simulink model "UnrealSimulinkController"  (R2025b)
settings: Solver=VariableStepAuto  StartTime=0.0  StopTime=inf  RelTol=1e-3
libraries: sim3dlib x3
settings Model: Creator=Liam  LastModifiedBy=Liam

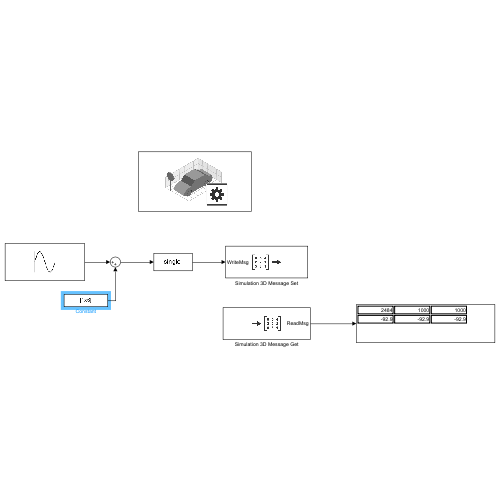
[thumbnail: Simulink's stored preview of the top-level diagram]
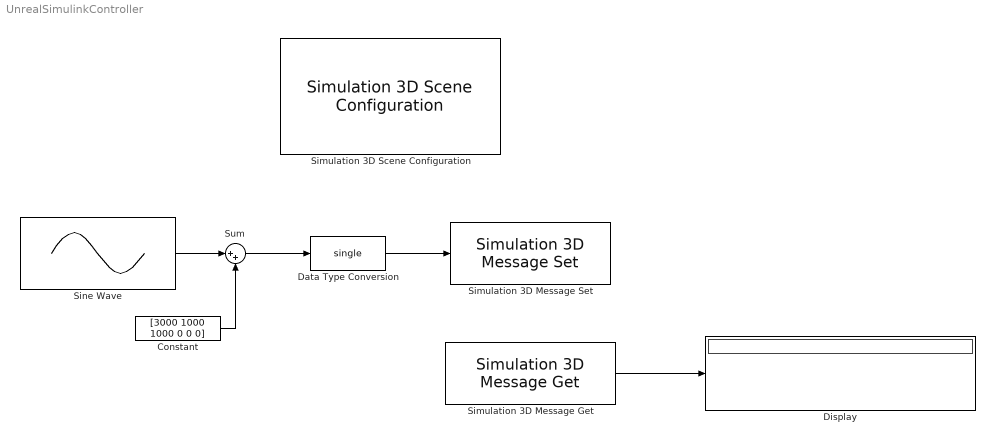
== system UnrealSimulinkController ==
  Constant : Constant  Value=[3000 1000 1000 0 0 0]  VectorParams1D=off  OutDataTypeStr=single
  Data Type Conversion : DataTypeConversion  OutDataTypeStr=single  SaturateOnIntegerOverflow=off  RndMeth=Floor
  Display : Display
  Simulation 3D Message Get : sim3dlib/Simulation 3D Message Get  Priority=1  SigName=ManateePoseGet  DataType=single  MsgSize=[1 6]  Ts=-1  aMode=0
      settings: LibrarySourceBlock=aerolibsim3d/Simulation 3D Message Get
  Simulation 3D Message Set : sim3dlib/Simulation 3D Message Set  Priority=-1  SigName=ManateePoseSet  Ts=-1  aMode=0
      settings: LibrarySourceBlock=aerolibsim3d/Simulation 3D Message Set
  Simulation 3D Scene Configuration : sim3dlib/Simulation 3D Scene Configuration  Priority=0  ProjectFormat=Unreal Editor  SceneDesc=Straight road  ProjectName=C:\Program Files\MATLAB\R2025b\toolbox\shared\sim3d_projects\automotive_project_windows\UE\WindowsNoEditor\VehicleSimulation.exe  ScenePath=/Game/Maps/HwStrght  UEProjPath=C:\Users\Liam\OneDrive\Documents\GitHub\Unreal_Simulink-Projects\SimulinkUnrealPluginTutorial\UnrealEnvironment\UnrealEnvironment.uproject  EnableOpenDRIVE=off  vehTagList={'Custom';'Scene Origin'}  vehTag=Scene Origin  AttachedCameraRelativeTranslation=[0 0 0]  FreeCameraDefaultInitialTranslation=[-6, 0, 2]  AttachedCameraRelativeRotation=[0 0 0]  FreeCameraDefaultInitialRotation=[0, -15, 0]  ViewpointName=Custom  FreeCameraInitialTranslation=[0, 0, 0]  ViewpointTranslation=[0 0 0]  FreeCameraInitialRotation=[0, 0, 0]  ViewpointRotation=[0 0 0]  OpVisEn=off  Ts=1/60  EnableWindow=on  EnableRemoteAccess=off  EnableWeather=off  SunAzimuth=90  SunAltitude=40.0  EnableGeospatialSun=off  Latitude=0  Longitude=0  Date=2023-01-01  Time=10:30:00  GeoTimeZone=-5.0  SunDaylightSaving=off  wind=1  clouds=10  EnableVolumetricClouds=off  CloudCoverage=0  CloudAltitude=6  fog=0  rain=0  RaindropsEffect=off  SnowDensity=0  EnableGeospatial=off  TilesetSource=Earth terrain  UseTrueOrigin=off  OriginHeight=200  OriginLatitude=40.744652  OriginLongitude=-73.988864  MapStyle=Aerial  AdditionalAssetIDs=[]  UseAdvancedSunSky=off  SolarTime=11  TimeZone=-5  Day=21  Month=9  Year=2022  UseDaylightSavingTime=on  DSTStartDay=10  DSTStartMonth=3  DSTEndDay=3  DSTEndMonth=11  DSTSwitchHour=2  sensorTag=MainCamera1  sensorId=1  sensorName=MainCamera1  mountLoc=Origin  offsetFlag=off  tmountOffset=[0, 0, 0]  rmountOffset=[0, 0, 0]  HorizontalResolution=1280  VerticalResolution=720  HorizontalFOV=60  mountPoint=[0 0 0]  mountOrientation=[0 0 0]  aMode=3  ID=1  GeoTrigger=Inactive  ViewNameList={'Custom'}  ViewTranslationList={'[0 0 0]'}  ViewRotationList={'[0 0 0]'}
      settings: LibrarySourceBlock=drivingsim3d/Simulation 3D Scene Configuration
  Sine Wave : Sin  Amplitude=[1000 0 0 180 180 180]  Frequency=[1,2,3,4,5,6]  SampleTime=0
  Sum : Sum  Inputs=|++
  wires:
  Constant/1 -> Sum/2
  Data Type Conversion/1 -> Simulation 3D Message Set/1
  Sine Wave/1 -> Sum/1
  Simulation 3D Message Get/1 -> Display/1
  Sum/1 -> Data Type Conversion/1
